simulink model "Modelo_NL_desacoplado_linealizado"  (R2021a)
settings: Solver=VariableStepAuto  StartTime=0.0  StopTime=10.0  RelTol=1e-3
undefined symbols (not defined in the file): alpha_cu, beq, Cts, g, Jeq, l_cm, l_l, lambda_m, Ld, Lls, Lq, m, m_l, Pp, r, Rs, Rs_REF, Rts_amb, Ts_REF
settings Model: Creator=fhlla  LastModifiedBy=fhlla

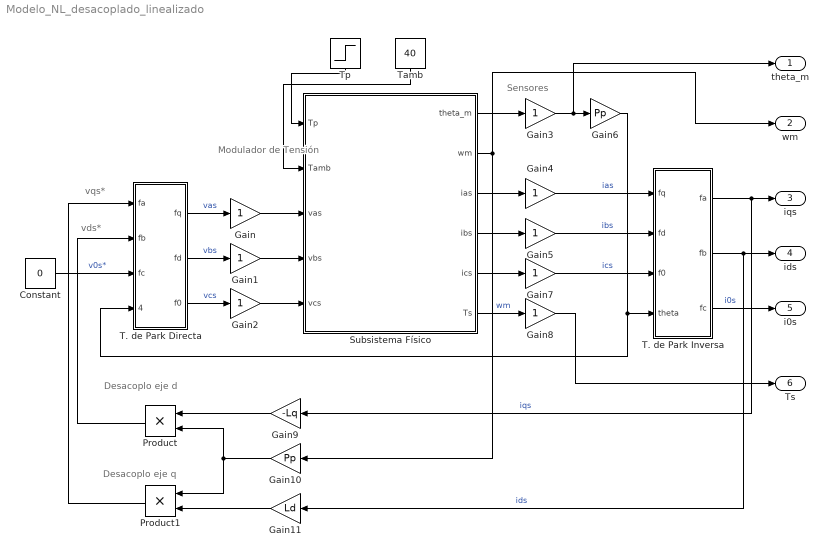
== system Modelo_NL_desacoplado_linealizado ==
  note: Desacoplo eje q
  note: Desacoplo eje d
  note: Modulador
      | de
      | Tensión
  note: Sensores
  note: vds*
  note: vqs*
  Constant : Constant  Value=0
  Gain{,1..5,7..8} (8 alike) : Gain
  Gain10 : Gain  Gain=Pp
  Gain11 : Gain  Gain=Ld
  Gain6 : Gain  Gain=Pp
  Gain9 : Gain  Gain=-Lq
  Product : Product
  Product1 : Product
  Subsistema Físico : Subsystem
  T. de Park Directa : MATLAB Function  TreatAsAtomicUnit=on
  T. de Park Inversa : MATLAB Function  TreatAsAtomicUnit=on
  Tamb : Constant  Value=40
  Tp : Step  SampleTime=0
  theta_m : Outport
  wm : Outport  Port=2
  iqs : Outport  Port=3
  ids : Outport  Port=4
  i0s : Outport  Port=5
  Ts : Outport  Port=6
  wires:
  Gain3/1 -> Gain6/1, theta_m/1
  Gain6/1 -> T. de Park Directa/4(theta_r), T. de Park Inversa/4(theta)
  Gain4/1 -> T. de Park Inversa/1(fq)  "ias"
  Gain5/1 -> T. de Park Inversa/2(fd)  "ibs"
  Subsistema Físico/5(ics) -> Gain7/1
  Subsistema Físico/4(ibs) -> Gain5/1
  Subsistema Físico/3(ias) -> Gain4/1
  Gain7/1 -> T. de Park Inversa/3(f0)  "ics"
  Subsistema Físico/1(theta_m) -> Gain3/1
  T. de Park Directa/1(fq) -> Gain/1  "vas"
  T. de Park Directa/2(fd) -> Gain1/1  "vbs"
  T. de Park Directa/3(f0) -> Gain2/1  "vcs"
  Gain/1 -> Subsistema Físico/3("vas ")
  Gain1/1 -> Subsistema Físico/4("vbs ")
  Gain2/1 -> Subsistema Físico/5("vcs ")
  Constant/1 -> T. de Park Directa/3(fc)  "v0s*"
  Tamb/1 -> Subsistema Físico/2(Tamb)
  Subsistema Físico/2(wm) -> Gain10/1, wm/1  "wm"
  T. de Park Inversa/1(fa) -> iqs/1, Gain9/1  "iqs"
  T. de Park Inversa/2(fb) -> Gain11/1, ids/1  "ids"
  T. de Park Inversa/3(fc) -> i0s/1  "i0s"
  Subsistema Físico/6(Ts) -> Gain8/1
  Gain8/1 -> Ts/1
  Product/1 -> T. de Park Directa/2(fb)
  Product1/1 -> T. de Park Directa/1(fa)
  Gain9/1 -> Product/1
  Gain11/1 -> Product1/2
  Gain10/1 -> Product1/1, Product/2
  Tp/1 -> Subsistema Físico/1(Tp)

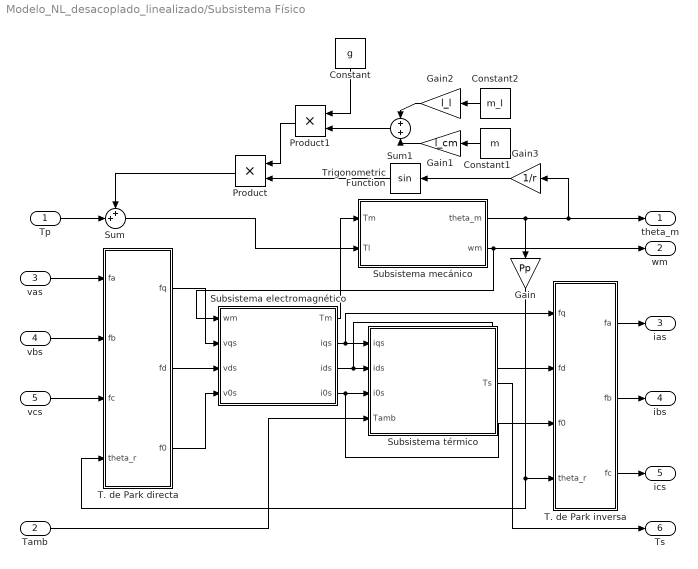
== system Modelo_NL_desacoplado_linealizado/Subsistema Físico ==
  Tp : Inport
  Tamb : Inport  Port=2
  "vas " : Inport  Port=3
  "vbs " : Inport  Port=4
  "vcs " : Inport  Port=5
  Constant : Constant  Value=g
  Constant1 : Constant  Value=m
  Constant2 : Constant  Value=m_l
  Gain : Gain  Gain=Pp
  Gain1 : Gain  Gain=l_cm
  Gain2 : Gain  Gain=l_l
  Gain3 : Gain  Gain=1/r
  Product : Product
  Product1 : Product
  Subsistema electromagnético : Subsystem
  Subsistema mecánico : Subsystem
  Subsistema térmico : Subsystem
  Sum : Sum  Inputs=++|
  Sum1 : Sum  Inputs=+|+
  T. de Park directa : Subsystem
  T. de Park inversa : Subsystem
  Trigonometric Function : Trigonometry
  theta_m : Outport
  wm : Outport  Port=2
  ias : Outport  Port=3
  ibs : Outport  Port=4
  ics : Outport  Port=5
  Ts : Outport  Port=6
  wires:
  Sum1/1 -> Product1/2
  Subsistema electromagnético/4(i0s) -> T. de Park inversa/3(f0), Subsistema térmico/3(i0s)
  Subsistema térmico/1(Ts) -> Ts/1
  Subsistema electromagnético/1(Tm) -> Subsistema mecánico/1(Tm)
  T. de Park inversa/2(fb) -> ibs/1
  "vas "/1 -> T. de Park directa/1("fa ")
  Subsistema electromagnético/3(ids) -> T. de Park inversa/2(fd), Subsistema térmico/2(ids)
  T. de Park directa/3(f0) -> Subsistema electromagnético/4(v0s)
  Tp/1 -> Sum/2
  T. de Park directa/2(fd) -> Subsistema electromagnético/3(vds)
  Product/1 -> Sum/1
  Tamb/1 -> Subsistema térmico/4(Tamb)
  Constant2/1 -> Gain2/1
  T. de Park inversa/1(fa) -> ias/1
  Trigonometric Function/1 -> Product/2
  "vbs "/1 -> T. de Park directa/2("fb ")
  Subsistema electromagnético/2(iqs) -> T. de Park inversa/1(fq), Subsistema térmico/1(iqs)
  Gain3/1 -> Trigonometric Function/1
  Gain/1 -> T. de Park directa/4(theta_r), T. de Park inversa/4(theta_r)
  Constant1/1 -> Gain1/1
  "vcs "/1 -> T. de Park directa/3("fc ")
  Constant/1 -> Product1/1
  Subsistema mecánico/1(theta_m) -> Gain/1, Gain3/1, theta_m/1
  T. de Park inversa/3(fc) -> ics/1
  T. de Park directa/1(fq) -> Subsistema electromagnético/2(vqs)
  Gain2/1 -> Sum1/1
  Gain1/1 -> Sum1/2
  Subsistema mecánico/2(wm) -> wm/1, Subsistema electromagnético/1(wm)
  Product1/1 -> Product/1
  Sum/1 -> Subsistema mecánico/2(Tl)

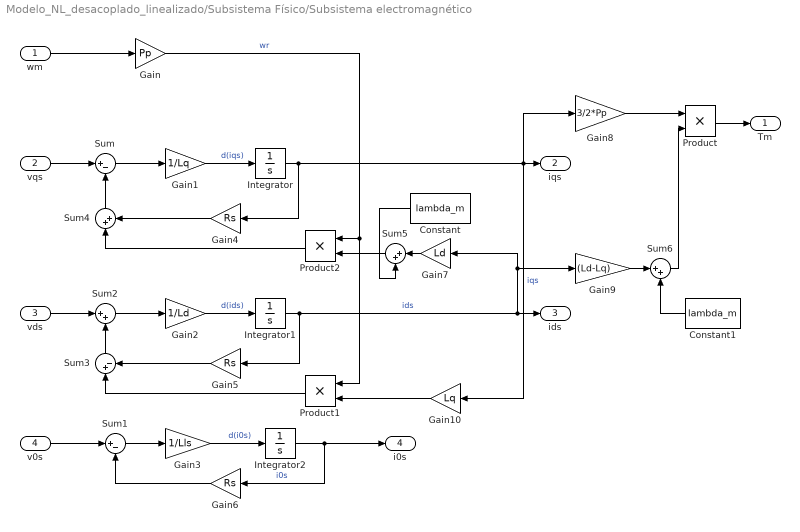
== system Modelo_NL_desacoplado_linealizado/Subsistema Físico/Subsistema electromagnético ==
  wm : Inport
  vqs : Inport  Port=2
  vds : Inport  Port=3
  v0s : Inport  Port=4
  Constant : Constant  Value=lambda_m
  Constant1 : Constant  Value=lambda_m
  Gain : Gain  Gain=Pp
  Gain1 : Gain  Gain=1/Lq
  Gain10 : Gain  Gain=Lq
  Gain2 : Gain  Gain=1/Ld
  Gain3 : Gain  Gain=1/Lls
  Gain4 : Gain  Gain=Rs
  Gain5 : Gain  Gain=Rs
  Gain6 : Gain  Gain=Rs
  Gain7 : Gain  Gain=Ld
  Gain8 : Gain  Gain=3/2*Pp
  Gain9 : Gain  Gain=(Ld-Lq)
  Integrator : Integrator
  Integrator1 : Integrator
  Integrator2 : Integrator
  Product : Product
  Product1 : Product
  Product2 : Product
  Sum : Sum  Inputs=|+-
  Sum1 : Sum  Inputs=|+-
  Sum{2,4..6} (4 alike) : Sum  Inputs=|++
  Sum3 : Sum  Inputs=|+-
  Tm : Outport
  iqs : Outport  Port=2
  ids : Outport  Port=3
  i0s : Outport  Port=4
  wires:
  Gain7/1 -> Sum5/1
  Sum1/1 -> Gain3/1
  Integrator1/1 -> Gain5/1, Gain9/1, Gain7/1, ids/1  "ids"
  Gain6/1 -> Sum1/2
  Gain/1 -> Product2/1, Product1/1  "wr"
  Product/1 -> Tm/1
  v0s/1 -> Sum1/1
  Gain9/1 -> Sum6/1
  Sum4/1 -> Sum/2
  Gain8/1 -> Product/1
  Sum5/1 -> Product2/2
  Gain1/1 -> Integrator/1  "d(iqs)"
  Constant/1 -> Sum5/2
  Integrator2/1 -> Gain6/1, i0s/1  "i0s"
  Gain10/1 -> Product1/2
  Sum/1 -> Gain1/1
  Product2/1 -> Sum4/1
  Integrator/1 -> Gain4/1, Gain10/1, Gain8/1, iqs/1  "iqs"
  vds/1 -> Sum2/1
  Constant1/1 -> Sum6/2
  Gain2/1 -> Integrator1/1  "d(ids)"
  Gain3/1 -> Integrator2/1  "d(i0s)"
  Product1/1 -> Sum3/1
  Sum2/1 -> Gain2/1
  Gain4/1 -> Sum4/2
  Sum3/1 -> Sum2/2
  vqs/1 -> Sum/1
  Sum6/1 -> Product/2
  wm/1 -> Gain/1
  Gain5/1 -> Sum3/2

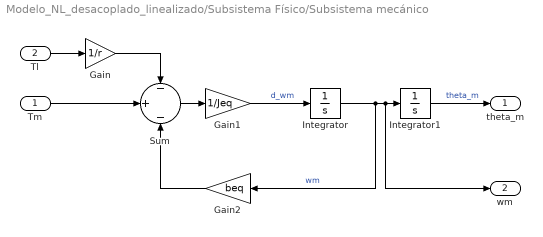
== system Modelo_NL_desacoplado_linealizado/Subsistema Físico/Subsistema mecánico ==
  Tm : Inport
  Tl : Inport  Port=2
  Gain : Gain  Gain=1/r
  Gain1 : Gain  Gain=1/Jeq
  Gain2 : Gain  Gain=beq
  Integrator : Integrator
  Integrator1 : Integrator
  Sum : Sum  Inputs=-|+|-
  theta_m : Outport
  wm : Outport  Port=2
  wires:
  Integrator1/1 -> theta_m/1  "theta_m"
  Tl/1 -> Gain/1
  Gain/1 -> Sum/1
  Sum/1 -> Gain1/1
  Gain1/1 -> Integrator/1  "d_wm"
  Tm/1 -> Sum/2
  Gain2/1 -> Sum/3
  Integrator/1 -> Gain2/1, wm/1, Integrator1/1  "wm"

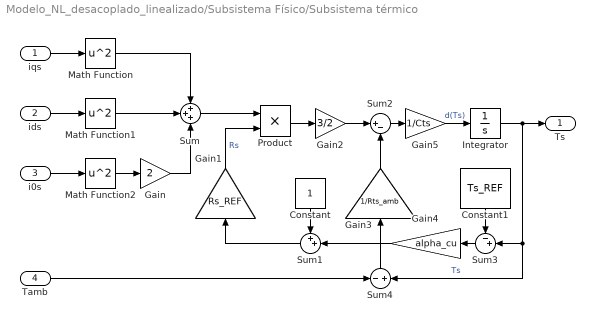
== system Modelo_NL_desacoplado_linealizado/Subsistema Físico/Subsistema térmico ==
  iqs : Inport
  ids : Inport  Port=2
  i0s : Inport  Port=3
  Tamb : Inport  Port=4
  Constant : Constant
  Constant1 : Constant  Value=Ts_REF
  Gain : Gain  Gain=2
  Gain1 : Gain  Gain=Rs_REF
  Gain2 : Gain  Gain=3/2
  Gain3 : Gain  Gain=1/Rts_amb
  Gain4 : Gain  Gain=alpha_cu
  Gain5 : Gain  Gain=1/Cts
  Integrator : Integrator
  Math Function : Math  Operator=square  SaturateOnIntegerOverflow=on
  Math Function1 : Math  Operator=square  SaturateOnIntegerOverflow=on
  Math Function2 : Math  Operator=square  SaturateOnIntegerOverflow=on
  Product : Product
  Sum : Sum  Inputs=+++
  Sum1 : Sum  Inputs=++|
  Sum2 : Sum  Inputs=|+-
  Sum3 : Sum  Inputs=-+|
  Sum4 : Sum  Inputs=-|+
  Ts : Outport
  wires:
  Sum/1 -> Product/1
  Tamb/1 -> Sum4/1
  Gain3/1 -> Sum2/2
  Sum1/1 -> Gain1/1
  Product/1 -> Gain2/1
  Integrator/1 -> Sum3/2, Sum4/2, Ts/1  "Ts"
  iqs/1 -> Math Function/1
  Gain5/1 -> Integrator/1  "d(Ts)"
  Sum2/1 -> Gain5/1
  Gain1/1 -> Product/2  "Rs"
  Constant/1 -> Sum1/1
  Gain/1 -> Sum/3
  ids/1 -> Math Function1/1
  i0s/1 -> Math Function2/1
  Gain2/1 -> Sum2/1
  Math Function1/1 -> Sum/2
  Sum4/1 -> Gain3/1
  Math Function2/1 -> Gain/1
  Math Function/1 -> Sum/1
  Constant1/1 -> Sum3/1
  Gain4/1 -> Sum1/2
  Sum3/1 -> Gain4/1

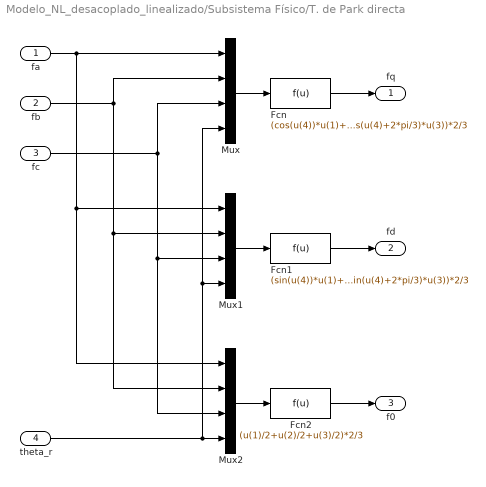
== system Modelo_NL_desacoplado_linealizado/Subsistema Físico/T. de Park directa ==
  "fa " : Inport
  "fb " : Inport  Port=2
  "fc " : Inport  Port=3
  theta_r : Inport  Port=4
  Fcn : Fcn  Expr=(cos(u(4))*u(1)+cos(u(4)-2*pi/3)*u(2)+cos(u(4)+2*pi/3)*u(3))*2/3
  Fcn1 : Fcn  Expr=(sin(u(4))*u(1)+sin(u(4)-2*pi/3)*u(2)+sin(u(4)+2*pi/3)*u(3))*2/3
  Fcn2 : Fcn  Expr=(u(1)/2+u(2)/2+u(3)/2)*2/3
  Mux : Mux
  Mux1 : Mux
  Mux2 : Mux
  fq : Outport
  fd : Outport  Port=2
  f0 : Outport  Port=3
  wires:
  Fcn2/1 -> f0/1
  Mux/1 -> Fcn/1
  "fc "/1 -> Mux1/3, Mux2/3, Mux/3
  "fa "/1 -> Mux/1, Mux1/1, Mux2/1
  theta_r/1 -> Mux/4, Mux1/4, Mux2/4
  Fcn/1 -> fq/1
  Mux1/1 -> Fcn1/1
  "fb "/1 -> Mux1/2, Mux2/2, Mux/2
  Fcn1/1 -> fd/1
  Mux2/1 -> Fcn2/1

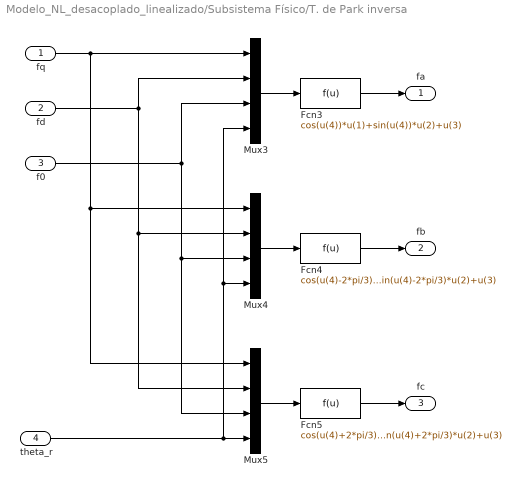
== system Modelo_NL_desacoplado_linealizado/Subsistema Físico/T. de Park inversa ==
  fq : Inport
  fd : Inport  Port=2
  f0 : Inport  Port=3
  theta_r : Inport  Port=4
  Fcn3 : Fcn  Expr=cos(u(4))*u(1)+sin(u(4))*u(2)+u(3)
  Fcn4 : Fcn  Expr=cos(u(4)-2*pi/3)*u(1)+sin(u(4)-2*pi/3)*u(2)+u(3)
  Fcn5 : Fcn  Expr=cos(u(4)+2*pi/3)*u(1)+sin(u(4)+2*pi/3)*u(2)+u(3)
  Mux3 : Mux
  Mux4 : Mux
  Mux5 : Mux
  fa : Outport
  fb : Outport  Port=2
  fc : Outport  Port=3
  wires:
  f0/1 -> Mux5/3, Mux4/3, Mux3/3
  Fcn3/1 -> fa/1
  fq/1 -> Mux3/1, Mux5/1, Mux4/1
  Mux5/1 -> Fcn5/1
  Mux4/1 -> Fcn4/1
  Mux3/1 -> Fcn3/1
  Fcn5/1 -> fc/1
  theta_r/1 -> Mux3/4, Mux4/4, Mux5/4
  Fcn4/1 -> fb/1
  fd/1 -> Mux5/2, Mux4/2, Mux3/2

== matlab function Modelo_NL_desacoplado_linealizado/T. de Park Inversa ==
  data: fq input; fa output; fd input; f0 input; theta input; fb output; fc output
function [fa,fb,fc] = TI_Park(fq,fd,f0,theta)
f = [        cos(theta)          sin(theta)        1;
     cos(theta - (2*pi)/3) sin(theta - (2*pi)/3)   1;
     cos(theta + (2*pi)/3) sin(theta + (2*pi)/3)   1];

resultados = f*[fq;fd;f0];
fa = resultados(1);
fb = resultados(2);
fc = resultados(3);

== matlab function Modelo_NL_desacoplado_linealizado/T. de Park Directa ==
  data: fa input; fq output; fb input; fc input; theta_r input; fd output; f0 output
function [fq, fd, f0] = TD_Park(fa, fb, fc, theta_r)
    f = (2/3) * [cos(theta_r)               cos(theta_r - (2*pi)/3)      cos(theta_r + (2*pi)/3);
                 sin(theta_r)               sin(theta_r - (2*pi)/3)      sin(theta_r + (2*pi)/3);
                 1/2                      1/2                        1/2                   ];

    resultados = f * [fa; fb; fc];
    fq = resultados(1);
    fd = resultados(2);
    f0 = resultados(3);
end
